simulink model "DDS_test"  (Simulink 9.1)
settings: Solver=VariableStepDiscrete  StartTime=0.0  StopTime=sim_time  RelTol=1e-3  EnableMultiTasking=on
values from neighbouring files (symbols this model uses):
  fclk = 100    [DDS_test_m.m]
  L = 15    [DDS_test_m.m]
  Pe = ((fo*(2^M))/fclk)/(2^M)    (= 0.01)    [DDS_test_m.m]
  W = 14    [DDS_test_m.m]
libraries: simulink x1
settings Model: Creator=jvalls  LastModifiedBy=jvalls
settings DataIOCC: LimitDataPoints=on
settings DebuggingCC: UnderspecifiedInitializationDetection=Simplified  MergeDetectMultiDrivingBlocksExec=error  SolverPrmCheckMsg=warning
settings GRTTargetCC: GeneratePreprocessorConditionals=Disable all  CombineOutputUpdateFcns=on  GRTInterface=off
settings ConfigComp: CovSFcnEnable=off

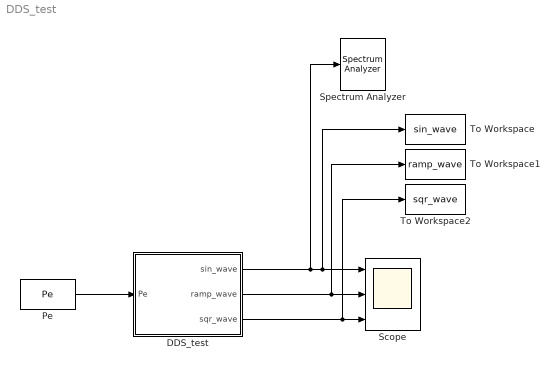
== system DDS_test ==
  DDS_test : Subsystem
  Pe : Constant  Value=Pe  SampleTime=1/fclk
  Scope : Scope  NumInputPorts=3
  Spectrum Analyzer : SpectrumAnalyzer
  To Workspace : ToWorkspace  VariableName=sin_wave  SampleTime=-1
      settings: Save2DSignal=2-D array (concatenate along first dimension)
  To Workspace1 : ToWorkspace  VariableName=ramp_wave  SampleTime=-1
      settings: Save2DSignal=2-D array (concatenate along first dimension)
  To Workspace2 : ToWorkspace  VariableName=sqr_wave  SampleTime=-1
      settings: Save2DSignal=2-D array (concatenate along first dimension)
  wires:
  Pe/1 -> DDS_test/1(Pe)
  DDS_test/2(ramp_wave) -> To Workspace1/1, Scope/2
  DDS_test/3(sqr_wave) -> To Workspace2/1, Scope/3
  DDS_test/1(sin_wave) -> Spectrum Analyzer/1, To Workspace/1, Scope/1

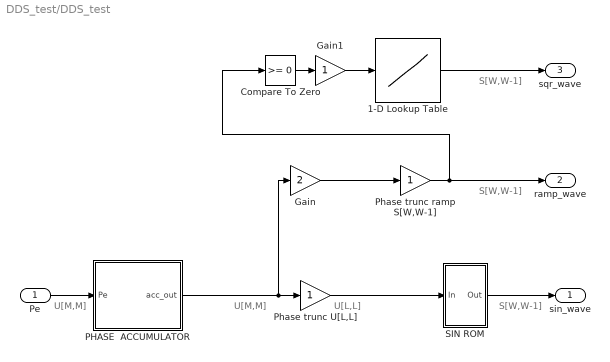
== system DDS_test/DDS_test ==
  note: S[W,W-1]
  note: S[W,W-1]
  note: S[W,W-1]
  note: U[M,M]
  note: U[L,L]
  note: U[M,M]
  Pe : Inport
  1-D Lookup Table : Lookup_n-D  NumberOfTableDimensions=1  BreakpointsForDimension1=[0:1]  Table=[ -1+2^-(W-1) 1-2^-(W-1)]  InternalRulePriority=Speed  RndMeth=Simplest  InputSameDT=on
  Compare To Zero : simulink/Logic and Bit Operations/Compare To Zero  relop=>=  OutDataTypeStr=boolean
  Gain : Gain  Gain=2
  Gain1 : Gain  OutDataTypeStr=double
  PHASE  ACCUMULATOR : Subsystem
  Phase trunc U[L,L] : Gain  OutDataTypeStr=fixdt(0,L,L)
  Phase trunc ramp S[W,W-1] : Gain  OutDataTypeStr=fixdt(1,W,W-1)
  SIN ROM : Subsystem
  sin_wave : Outport
  ramp_wave : Outport  Port=2
  sqr_wave : Outport  Port=3
  wires:
  Phase trunc U[L,L]/1 -> SIN ROM/1(In)
  SIN ROM/1(Out) -> sin_wave/1
  Pe/1 -> PHASE  ACCUMULATOR/1(Pe)
  Phase trunc ramp S[W,W-1]/1 -> Compare To Zero/1, ramp_wave/1
  1-D Lookup Table/1 -> sqr_wave/1
  Gain/1 -> Phase trunc ramp S[W,W-1]/1
  PHASE  ACCUMULATOR/1(acc_out) -> Phase trunc U[L,L]/1, Gain/1
  Gain1/1 -> 1-D Lookup Table/1
  Compare To Zero/1 -> Gain1/1

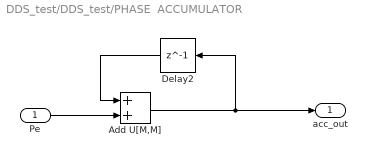
== system DDS_test/DDS_test/PHASE  ACCUMULATOR ==
  Pe : Inport
  Add U[M,M] : Sum  AccumDataTypeStr=fixdt(0,M,M)  OutDataTypeStr=fixdt(0,M,M)  RndMeth=Convergent
  Delay2 : Delay  DelayLength=1
  acc_out : Outport
  wires:
  Add U[M,M]/1 -> acc_out/1, Delay2/1
  Pe/1 -> Add U[M,M]/2
  Delay2/1 -> Add U[M,M]/1

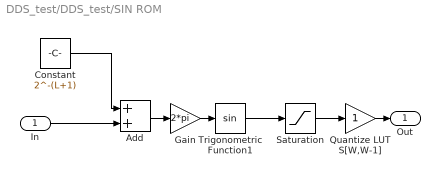
== system DDS_test/DDS_test/SIN ROM ==
  In : Inport
  Add : Sum
  Constant : Constant  Value=2^-(L+1)
  Gain : Gain  Gain=2*pi
  Quantize LUT S[W,W-1] : Gain  OutDataTypeStr=fixdt(1,W,W-1)  RndMeth=Round  SaturateOnIntegerOverflow=on
  Saturation : Saturate  UpperLimit=1-2^-(W-1)  LowerLimit=-(1-2^-(W-1))
  Trigonometric Function1 : Trigonometry
  Out : Outport
  wires:
  Add/1 -> Gain/1
  In/1 -> Add/2
  Constant/1 -> Add/1
  Quantize LUT S[W,W-1]/1 -> Out/1
  Trigonometric Function1/1 -> Saturation/1
  Gain/1 -> Trigonometric Function1/1
  Saturation/1 -> Quantize LUT S[W,W-1]/1
